simulink model "USBxiangyi"  (R2017b)
settings: Solver=VariableStepAuto  StartTime=0.0  StopTime=10.0  RelTol=1e-3
libraries: dsparch4 x2
settings Model: Creator=DELL  LastModifiedBy=DELL

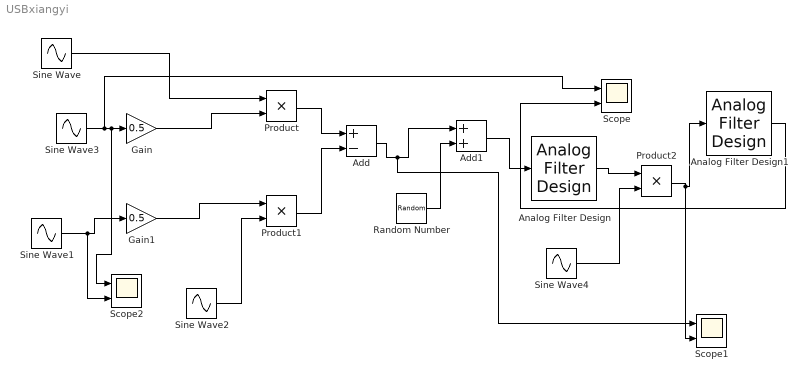
== system USBxiangyi ==
  Add : Sum  Inputs=+-
  Add1 : Sum
  Analog Filter Design : dsparch4/Analog Filter Design  method=Butterworth  filttype=Bandpass  N=8  Wlo=100  Whi=110  Rp=2  Rs=40
  Analog Filter Design1 : dsparch4/Analog Filter Design  method=Butterworth  filttype=Lowpass  N=8  Wlo=10  Whi=80  Rp=2  Rs=40
  Gain : Gain  Gain=0.5
  Gain1 : Gain  Gain=0.5
  Product : Product
  Product1 : Product
  Product2 : Product
  Random Number : RandomNumber  Variance=0.01  SampleTime=1
  Scope : Scope  NumInputPorts=2
  Scope1 : Scope  NumInputPorts=2
  Scope2 : Scope  NumInputPorts=2
  Sine Wave : Sin  Frequency=100  SampleTime=0
  Sine Wave1 : Sin  Frequency=10  SampleTime=0
  Sine Wave2 : Sin  Frequency=100  SampleTime=0
  Sine Wave3 : Sin  Frequency=10  Phase=3*pi/2  SampleTime=0
  Sine Wave4 : Sin  Frequency=100  SampleTime=0
  wires:
  Sine Wave3/1 -> Scope/1, Scope2/1, Gain/1
  Gain/1 -> Product/2
  Sine Wave/1 -> Product/1
  Sine Wave1/1 -> Scope2/2, Gain1/1
  Sine Wave2/1 -> Product1/2
  Gain1/1 -> Product1/1
  Product/1 -> Add/1
  Product1/1 -> Add/2
  Random Number/1 -> Add1/2
  Add1/1 -> Analog Filter Design/1
  Sine Wave4/1 -> Product2/2
  Analog Filter Design1/1 -> Scope/2
  Analog Filter Design/1 -> Product2/1
  Product2/1 -> Scope1/2, Analog Filter Design1/1
  Add/1 -> Scope1/1, Add1/1
